simulink model "thy"  (R2018a)
settings: Solver=VariableStepAuto  StartTime=0.0  StopTime=0.1  RelTol=1e-3
libraries: powerlib x11, powerlib_meascontrol x1
settings Model: Creator=pc  LastModifiedBy=pc

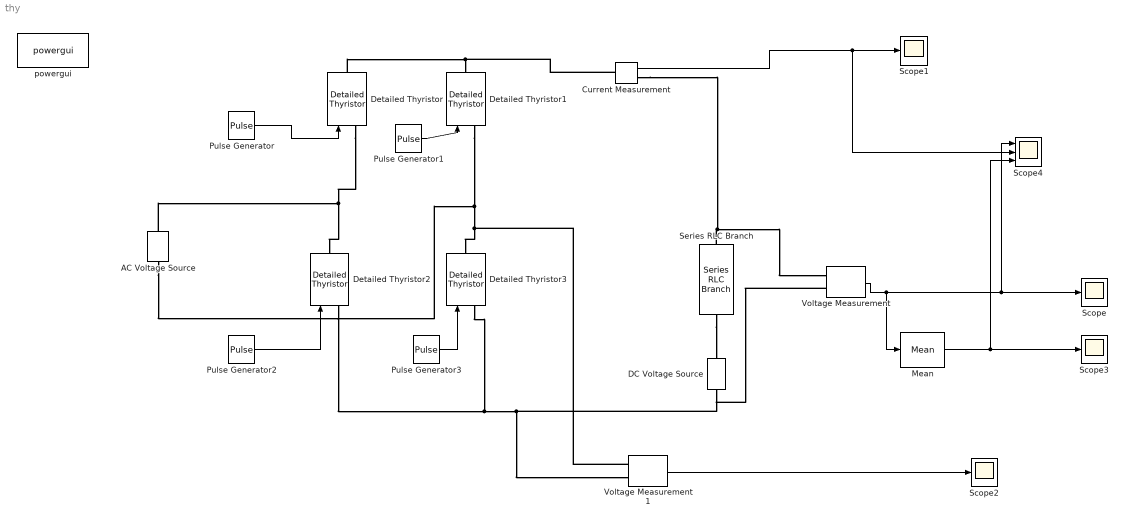
== system thy ==
  AC Voltage Source : powerlib/Electrical Sources/AC Voltage Source  Amplitude=100  Phase=0  Frequency=50  SampleTime=0  Measurements=None  BusType=swing  Pref=10e3  Qref=0  Qmin=-inf  Qmax=+inf
  Current Measurement : powerlib/Measurements/Current Measurement  PhasorSimulation=off  OutputType=Complex  PSBequivalent=0
  DC Voltage Source : powerlib/Electrical Sources/DC Voltage Source  Amplitude=20  Measurements=None
  Detailed Thyristor{,1..3} (4 alike) : powerlib/Power Electronics/Detailed Thyristor  Ron=0.001  Lon=1e-3  Vf=0  IL=0.1  Tq=100e-6  IC=0  Rs=500  Cs=250e-9  Measurements=off
      settings: SourceProductName=Simscape Power Systems  SourceProductBaseCode=PS
  Mean : powerlib_meascontrol/Measurements/Mean  Freq=50  Vinit=0  Ts=0
  Pulse Generator : DiscretePulseGenerator  PulseType=Time based  Period=0.02  PulseWidth=5  PhaseDelay=0.005
  Pulse Generator1 : DiscretePulseGenerator  PulseType=Time based  Period=0.02  PulseWidth=5  PhaseDelay=0.015
  Pulse Generator2 : DiscretePulseGenerator  PulseType=Time based  Period=0.02  PulseWidth=5  PhaseDelay=0.015  VectorParams1D=off
  Pulse Generator3 : DiscretePulseGenerator  PulseType=Time based  Period=0.02  PulseWidth=5  PhaseDelay=0.005
  Scope{,1..3} (4 alike) : Scope
  Scope4 : Scope  NumInputPorts=3
  Series RLC Branch : powerlib/Elements/Series RLC Branch  LConnTagsString=__new0  RConnTagsString=__new0  BranchType=RL  Resistance=10  Inductance=5e-3  SetiL0=off  InitialCurrent=0  Capacitance=1e-6  Setx0=off  InitialVoltage=0  Measurements=None
  Voltage Measurement : powerlib/Measurements/Voltage Measurement  PhasorSimulation=off  OutputType=Complex  PSBequivalent=0
  Voltage Measurement1 : powerlib/Measurements/Voltage Measurement  PhasorSimulation=off  OutputType=Complex  PSBequivalent=0
  powergui : powerlib/powergui  Priority=1  SimulationMode=Discrete  SampleTime=5e-6  frequency=60  Iterations=50  frequencyindice=50  Pbase=100e6  ErrMax=1e-4  UnitsV=kV  UnitsW=MW  buscounter=0  FunctionMessages=off  echomessages=off  EnableUseOfTLC=off  CurrentSourceSwitches=off  DisableSnubberDevices=off  DisableRonSwitches=off  DisableVfSwitches=off  DisplayEquations=off  SolverType=Tustin/Backward Euler (TBE)  Interpol=off  ExternalGateDelay=off  methode=off  Ts=100  x0status=blocks  SPID=on  SwTol=0  HookPort=off  RestoreLinks=warning  ResistiveCurrentMeasurement=off  Frange=[0:2:500]  Ylog=off  Xlog=on  ShowGrid=off  save=off  variable=ZData  structure=0  ZoomFFT=off  StartTime=0.0  cycles=1  DisplayStyle=1  fundamental=60  FreqAxis=off  MaxFrequency=1000  frequencyindicesteady=1  RmsSteady=1  display=off
  wires:
  Pulse Generator2/1 -> Detailed Thyristor2/1
  Pulse Generator3/1 -> Detailed Thyristor3/1
  Pulse Generator1/1 -> Detailed Thyristor1/1
  Pulse Generator/1 -> Detailed Thyristor/1
  Current Measurement/1 -> Scope4/2, Scope1/1
  Voltage Measurement1/1 -> Scope2/1
  Mean/1 -> Scope4/3, Scope3/1
  Voltage Measurement/1 -> Mean/1, Scope4/1, Scope/1
  connections:
  Detailed Thyristor2/LConn1 -- Detailed Thyristor3/LConn1 -- Voltage Measurement/LConn2 -- DC Voltage Source/LConn1 -- Voltage Measurement1/LConn2
  Detailed Thyristor/RConn1 -- Current Measurement/LConn1 -- Detailed Thyristor1/RConn1
  Detailed Thyristor/LConn1 -- AC Voltage Source/RConn1 -- Detailed Thyristor2/RConn1
  Detailed Thyristor1/LConn1 -- AC Voltage Source/LConn1 -- Voltage Measurement1/LConn1 -- Detailed Thyristor3/RConn1
  Series RLC Branch/LConn1 -- Current Measurement/RConn1 -- Voltage Measurement/LConn1
  Series RLC Branch/RConn1 -- DC Voltage Source/RConn1
